simulink model "OES_rel_YA"  (R2018b)
settings: configuration reference "Configuration" (kept outside this file)
undefined symbols (not defined in the file): sats, TimeStep
settings Model: Creator=Ethan  LastModifiedBy=Ethan
settings ConfigSetRef: SourceLocation=Base Workspace

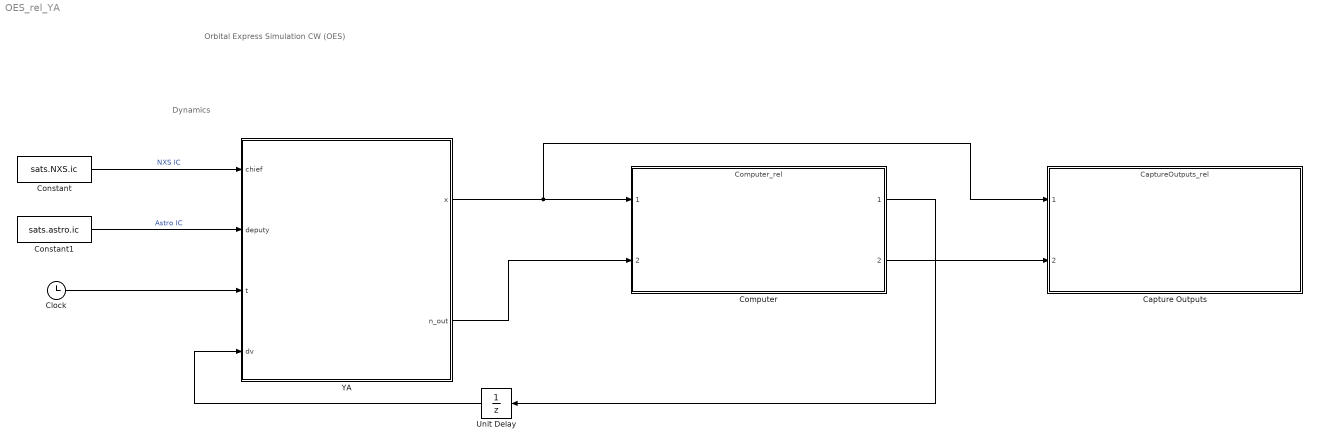
== system OES_rel_YA ==
  note: Dynamics
  note: Orbital Express Simulation CW (OES)
  Capture Outputs : ModelReference  ModelNameDialog=CaptureOutputs_rel.slx  ParameterArgumentNames=CON  ParameterArgumentValues=CON  UsingDefaultArgumentValue=0  SimulationMode=Normal  ModelReferenceVersion=1.61
  Clock : Clock
  Computer : ModelReference  ModelNameDialog=Computer_rel.slx  ParameterArgumentNames=CON  ParameterArgumentValues=CON  UsingDefaultArgumentValue=0  SimulationMode=Normal  ModelReferenceVersion=1.233
  Constant : Constant  Value=sats.NXS.ic  OutDataTypeStr=Bus: Bus_state
  Constant1 : Constant  Value=sats.astro.ic  OutDataTypeStr=Bus: Bus_state
  Unit Delay : UnitDelay  SampleTime=-1
  YA : MATLAB Function  TreatAsAtomicUnit=on  SystemSampleTime=TimeStep
  wires:
  Constant/1 -> YA/1(chief)  "NXS IC"
  Constant1/1 -> YA/2(deputy)  "Astro IC"
  Clock/1 -> YA/3(t)
  YA/1(x) -> Capture Outputs/1, Computer/1
  YA/2(n_out) -> Computer/2
  Computer/2 -> Capture Outputs/2
  Computer/1 -> Unit Delay/1
  Unit Delay/1 -> YA/4(dv)

== matlab function OES_rel_YA/YA ==
  data: chief input; x output; deputy input; t input; dv input; CON parameter; n_out output
function [x, n_out] = YA_prop(chief, deputy, t, dv,CON)
persistent x0 t0 x_prev h e n Ainv M0
if isempty(x0)
%     [rHill,vHill] = ECI2Hill_Vectorized(chief.r_i,chief.v_i, ...
%         deputy.r_i,deputy.v_i);
%     [T,~,~] = ECI2RSW(chief.r_i,chief.v_i);
%     rHill = T * (deputy.r_i - chief.r_i);
%     omega = cross(chief.r_i, chief.v_i) / norm(chief.r_i)^2;
%     dv = deputy.v_i - chief.v_i - cross(omega, rHill);
%     vHill = T * dv;
%     x0 = [rHill; vHill];
    x0 = [.100, .010, .010, 0.0001, 0.0001, 0.0001]';
    f0 = 45;
    e = 0.7;
%     [a, ~, ~, ~, ~, ~] = rvECI2oe(deputy.r_i,deputy.v_i, CON.mu);
    a = 22926;
    k = 1 + e * cosd(f0);
    x0 = x0 / k;
    n = sqrt(CON.mu / a^3);
    h = norm(cross(deputy.r_i, deputy.v_i));
    t0 = t;
    x_prev = x0;
%     Ainv = YAinv_state_matrix(f0, e);
    A = YA_state_matrix(f0 * pi / 180, e, CON.mu, h, 0);
    Ainv = inv(A);
    E0 = 2 * atan(sqrt((1-e)/(1+e)) * tand(f0/2));
    M0 = E0 - e * sin(E0);
end

M = M0 + n * (t - t0);
E = M2E(M, e, 1e-6);

f = 2 * atan(sqrt((1+e)/(1-e)) * tan(E/2));

[A, k] = YA_state_matrix(f, e, CON.mu, h, t-t0);

n_out = n;

if any(dv ~= zeros(3, 1))
    x0(4:6) = x_prev(4:6) + dv;
    x0(1:3) = x_prev(1:3);
    A = YA_state_matrix(f, e, CON.mu, h, 0);
    x = A * Ainv * x0 * k;
    t0 = t;
else
    x = A * Ainv * x0 * k;
end
x_prev = x;
end
